simulink model "fxpdemo_state_space"  (Simulink 7.6)
settings: Solver=ode5  SolverMode=SingleTasking  StartTime=0.0  StopTime=2  FixedStep=SampleTime/5  RelTol=1e-3  AbsTol=1e-6
PreLoadFcn:
  | preload_state_space
InitFcn:
  | ;
StartFcn:
  | ;
StopFcn:
  | ;
values from neighbouring files (symbols this model uses):
  SampleTime = 0.01    [preload_state_space.m]
  xb0_z = inv( eye(length(Ab_z)) - Ab_z ) * Bb_z * u0    [preload_state_space.m]
  xc0_s = inv( -Ac_s ) * Bc_s * u0    [preload_state_space.m]
  xc0_z = inv( eye(length(Ac_z)) - Ac_z ) * Bc_z * u0    [preload_state_space.m]
undefined symbols (not defined in the file or in its folder): Ab_z, Ac_s, Ac_z, Bb_z, Bc_s, Bc_z, Cb_z, Cc_s, Cc_z, Db_z, Dc_s, Dc_z
libraries: simulink x2
Description:
  | Fixed-Point State Space
  | 
  | Sample implementations of fixed-point state space realizations are presented with a
  | comparison to floating point implementations.
PreSaveFcn:
  | ;
CloseFcn:
  | close_state_space;
settings Model: MinMaxOverflowLogging=MinMaxAndOverflow  Creator=The MathWorks Inc.  CovMetricSettings=d  ExtModeTrigMode=oneshot  ExtModeArmWhenConnect=off  ExtModeAutoUpdateStatusClock=off
settings DataIOCC: LimitDataPoints=off  SignalLoggingName=sigsOut
settings OptimizationCC: InlineParams=on  InitFltsAndDblsToZero=on  EfficientMapNaN2IntZero=off
settings DebuggingCC: SaveWithParameterizedLinksMsg=none  SignalResolutionControl=TryResolveAllWithWarning  SolverPrmCheckMsg=none  MultiTaskDSMMsg=warning  MultiTaskCondExecSysMsg=none  SigSpecEnsureSampleTimeMsg=none  IntegerOverflowMsg=none  ParameterDowncastMsg=warning  ParameterOverflowMsg=warning  ParameterPrecisionLossMsg=none  StrictBusMsg=None
settings HardwareCC: TargetUnknown=on
settings RTWCC: GenerateReport=on  IncludeERTFirstTime=on
settings GRTTargetCC: TargetFcnLib=ansi_tfl_tmw.mat

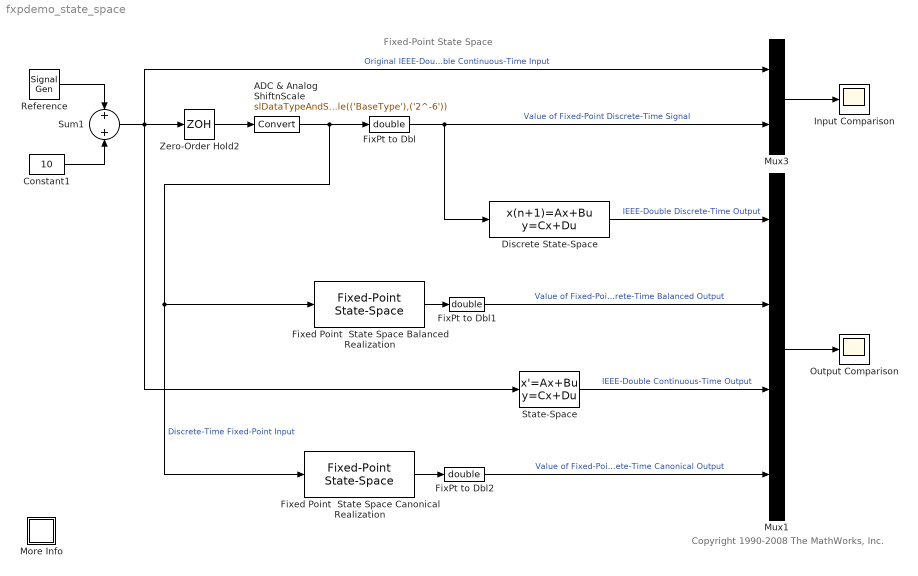
== system fxpdemo_state_space ==
  note: Copyright 1990-2008 The MathWorks, Inc.
  note: Fixed-Point State Space
  ADC & Analog ShiftnScale : DataTypeConversion  OutDataTypeStr=slDataTypeAndScale(('BaseType'),('2^-6'))  RndMeth=Nearest  SaturateOnIntegerOverflow=on  LockScale=on
  Constant1 : Constant  Value=10
  Discrete State-Space : DiscreteStateSpace  A=Ac_z  B=Bc_z  C=Cc_z  D=Dc_z  X0=xc0_z  SampleTime=SampleTime
  FixPt to Dbl : DataTypeConversion  OutDataTypeStr=double
  FixPt to Dbl1 : DataTypeConversion  OutDataTypeStr=double
  FixPt to Dbl2 : DataTypeConversion  OutDataTypeStr=double
  Fixed Point  State Space Balanced Realization : simulink/Additional Math & Discrete/Additional Discrete/Fixed-Point State-Space  SystemSampleTime=-1  A=Ab_z  B=Bb_z  C=Cb_z  D=Db_z  X0=xb0_z  InternalDataType=LongType  StateEqScaling=2^(-14)  OutputEqScaling=2^(-15)  DoSatur=off
  Fixed Point  State Space Canonical Realization : simulink/Additional Math & Discrete/Additional Discrete/Fixed-Point State-Space  SystemSampleTime=-1  A=Ac_z  B=Bc_z  C=Cc_z  D=Dc_z  X0=xc0_z  InternalDataType=LongType  StateEqScaling=2^(-12)  OutputEqScaling=2^(-15)  DoSatur=off
  Input Comparison : Scope
      settings: TickLabels=on  YMin=-10  YMax=30  SaveName=InputComparison
  More Info : Subsystem
      settings: OpenFcn=showdemo(bdroot(gcs))
      mask Display: disp('?')
  Mux1 : Mux
  Mux3 : Mux  Inputs=2
  Output Comparison : Scope
      settings: TickLabels=on  TimeRange=2  YMin=-60  YMax=140  SaveName=OutputComparison
  Reference : SignalGenerator  WaveForm=square  Amplitude=-10  Frequency=0.5
  State-Space : StateSpace  A=Ac_s  B=Bc_s  C=Cc_s  D=Dc_s  X0=xc0_s
  Sum1 : Sum  Inputs=2  SaturateOnIntegerOverflow=on  InputSameDT=on  OutDataTypeStr=Inherit: Same as first input
  Zero-Order Hold2 : ZeroOrderHold  SampleTime=SampleTime
  wires:
  Reference/1 -> Sum1/1
  Constant1/1 -> Sum1/2
  Sum1/1 -> Mux3/1, State-Space/1, Zero-Order Hold2/1  "Original IEEE-Double Continuous-Time Input"
  Zero-Order Hold2/1 -> ADC & Analog ShiftnScale/1
  ADC & Analog ShiftnScale/1 -> FixPt to Dbl/1, Fixed Point  State Space Balanced Realization/1, Fixed Point  State Space Canonical Realization/1  "Discrete-Time Fixed-Point Input"
  FixPt to Dbl/1 -> Mux3/2, Discrete State-Space/1  "Value of Fixed-Point Discrete-Time Signal"
  Fixed Point  State Space Canonical Realization/1 -> FixPt to Dbl2/1
  FixPt to Dbl1/1 -> Mux1/2  "Value of Fixed-Point Discrete-Time Balanced Output"
  Fixed Point  State Space Balanced Realization/1 -> FixPt to Dbl1/1
  State-Space/1 -> Mux1/3  "IEEE-Double Continuous-Time Output"
  Discrete State-Space/1 -> Mux1/1  "IEEE-Double Discrete-Time Output"
  FixPt to Dbl2/1 -> Mux1/4  "Value of Fixed-Point Discrete-Time Canonical Output"
  Mux1/1 -> Output Comparison/1
  Mux3/1 -> Input Comparison/1

== system fxpdemo_state_space/More Info ==
